simulink model "MATE_SynchronousMachine"  (R2024b)
settings: Solver=FixedStepDiscrete  StartTime=0.0  StopTime=6  FixedStep=Ts  RelTol=1e-4  EnableMultiTasking=on
PostLoadFcn:
  | Ts=25e-6;offset=4;
InitFcn:
  | Ts=25e-6;offset=4;
undefined symbols (not defined in the file): DiscIntNeverNeededParam, MATE, Phase, Rsnu, Single
libraries: fl_lib x58, nesl_utility x43, ee_lib x13, simetran x5, simetranss x3, powerlib_extras x3, simulink_extras x2, simulink x2
(part 2 of 4)

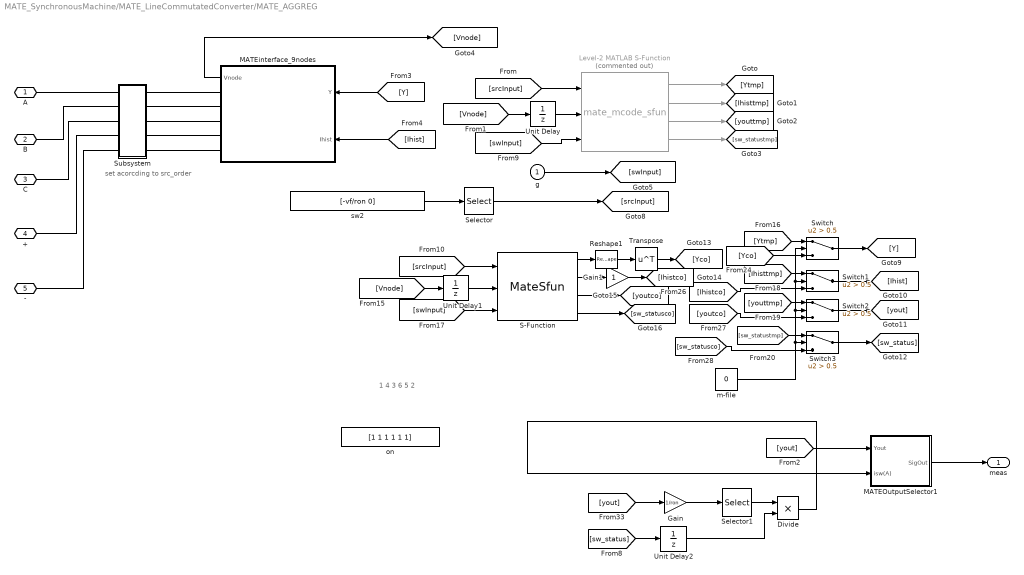
== system MATE_SynchronousMachine/MATE_LineCommutatedConverter/MATE_AGGREG ==
  note: set acorcding to src_order
  note: 1 4 3 6 5 2
  g : Inport
  Divide : Product
  Gain : Gain  Gain=1/ron
  Gain1 : Gain
  Level-2 MATLAB S-Function : M-S-Function  Commented=on  FunctionName=mate_mcode_sfun  Parameters=MATE,vf
  MATEOutputSelector1 : Subsystem
  MATEinterface_9nodes : Subsystem
  Reshape1 : Reshape  OutputDimensionality=Customize  OutputDimensions=[MATE.NumberOfNodes,MATE.NumberOfNodes]
  S-Function : S-Function  FunctionName=MateSfun  Parameters="MATERT.sizes,MATERT.As  ,MATERT.Bs,MATERT.Cs,MATERT.Ds,MATERT.Rsw,MATERT.SwType,MATERT.DISC,MATERT.h,MATERT.U0,MATERT.X0,vf"  SFunctionDeploymentMode=off  EnableBusSupport=off
  Selector : Selector  InputPortWidth=2  IndexOptions=Index vector (dialog)  Indices="[1 1 1 1 1 1  2 2 2 2 2]"  OutputSizes=1
  Selector1 : Selector  InputPortWidth=11  IndexOptions=Index vector (dialog)  Indices=[1 2 3 4 5 6]  OutputSizes=1
  Subsystem : Subsystem
  Switch{,1..3} (4 alike) : Switch  Criteria=u2 > Threshold  Threshold=0.5  SaturateOnIntegerOverflow=off  InputSameDT=off
  Transpose : Math  Operator=transpose
  Unit Delay : UnitDelay  SampleTime=Ts  HasFrameUpgradeWarning=on
  Unit Delay1 : UnitDelay  SampleTime=Ts  HasFrameUpgradeWarning=on
  Unit Delay2 : UnitDelay  SampleTime=Ts  HasFrameUpgradeWarning=on
  m-file : Constant  Value=0
  on : Constant  Value=[1 1 1 1 1 1]
  sw2 : Constant  Value=[-vf/ron 0]
  A : PMIOPort  Side=Left
  B : PMIOPort  Port=2  Side=Left
  C : PMIOPort  Port=3  Side=Left
  + : PMIOPort  Port=4  Side=Right
  - : PMIOPort  Port=5  Side=Right
  meas : Outport
  wires:
  m-file/1 -> Switch3/2, Switch/2, Switch1/2, Switch2/2
  Level-2 MATLAB S-Function/1 -> [Ytmp]
  Unit Delay/1 -> Level-2 MATLAB S-Function/2
  [swInput] -> S-Function/3
  S-Function/3 -> [youtco]
  Level-2 MATLAB S-Function/2 -> [Ihisttmp]
  Level-2 MATLAB S-Function/3 -> [youttmp]
  [youtco] -> Switch2/3
  [sw_statustmp] -> Switch3/1
  [Vnode] -> Unit Delay1/1
  [youttmp] -> Switch2/1
  [srcInput] -> Level-2 MATLAB S-Function/1
  Gain1/1 -> [Ihistco]
  [Ihistco] -> Switch1/3
  [Ytmp] -> Switch/1
  [Ihist] -> MATEinterface_9nodes/2(Ihist)
  [Vnode] -> Unit Delay/1
  [srcInput] -> S-Function/1
  Unit Delay1/1 -> S-Function/2
  S-Function/1 -> Reshape1/1
  S-Function/2 -> Gain1/1
  Switch2/1 -> [yout]
  Transpose/1 -> [Yco]
  Reshape1/1 -> Transpose/1
  S-Function/4 -> [sw_statusco]
  Switch/1 -> [Y]
  [Ihisttmp] -> Switch1/1
  [sw_statusco] -> Switch3/3
  MATEinterface_9nodes/1(Vnode) -> [Vnode]
  [swInput] -> Level-2 MATLAB S-Function/3
  [Yco] -> Switch/3
  Switch1/1 -> [Ihist]
  [Y] -> MATEinterface_9nodes/1(Y)
  Switch3/1 -> [sw_status]
  Level-2 MATLAB S-Function/4 -> [sw_statustmp]
  sw2/1 -> Selector/1
  Selector/1 -> [srcInput]
  Divide/1 -> MATEOutputSelector1/2(isw(A))
  Selector1/1 -> Divide/1
  [sw_status] -> Unit Delay2/1
  [yout] -> MATEOutputSelector1/1(Yout)
  Gain/1 -> Selector1/1
  Unit Delay2/1 -> Divide/2
  [yout] -> Gain/1
  MATEOutputSelector1/1(SigOut) -> meas/1
  g/1 -> [swInput]
  connections:
  Subsystem/RConn1 -- MATEinterface_9nodes/RConn1
  B/RConn1 -- Subsystem/LConn2
  A/RConn1 -- Subsystem/LConn1
  C/RConn1 -- Subsystem/LConn3
  +/RConn1 -- Subsystem/LConn4
  -/RConn1 -- Subsystem/LConn5
  Subsystem/RConn2 -- MATEinterface_9nodes/RConn2
  Subsystem/RConn3 -- MATEinterface_9nodes/RConn3
  Subsystem/RConn4 -- MATEinterface_9nodes/RConn4
  Subsystem/RConn5 -- MATEinterface_9nodes/RConn5

== system MATE_SynchronousMachine/Mesure et visualisation/Discrete Mean value ==
  In : Inport
  Constant : Constant  Value=Vinit  SampleTime=Ts
  Discrete Variable Transport Delay : powerlib_extras/Discrete  Control Blocks/Discrete Variable Transport Delay  MaxDelay=Delay+Ts  InitialValue=0  Ts=Ts
  Gain : Gain  Gain=K1  SaturateOnIntegerOverflow=on  OutDataTypeStr=Inherit: Same as input  ParamDataTypeStr=Inherit: Same as input
  Gain1 : Gain  Gain=K2  SaturateOnIntegerOverflow=on  OutDataTypeStr=Inherit: Same as input  ParamDataTypeStr=Inherit: Same as input
  Integ4 : DiscreteIntegrator  IntegratorMethod=Integration: Trapezoidal  SampleTime=Ts  ICPrevOutput=DiscIntNeverNeededParam  ICPrevScaledInput=DiscIntNeverNeededParam
  K1 : Constant  Value=Delay  SampleTime=Ts
  K2 : Constant  Value=Freq  SampleTime=Ts
  Product : Product  InputSameDT=on  SaturateOnIntegerOverflow=on  OutDataTypeStr=Inherit: Same as first input
  Step : Step  Time=1/Freq  SampleTime=Ts
  Sum1 : Sum  Inputs=+-  InputSameDT=on  SaturateOnIntegerOverflow=on  OutDataTypeStr=Inherit: Same as first input
  Sum5 : Sum  InputSameDT=on  SaturateOnIntegerOverflow=on  OutDataTypeStr=Inherit: Same as first input
  Sum7 : Sum  Inputs=-+  InputSameDT=on  SaturateOnIntegerOverflow=on  OutDataTypeStr=Inherit: Same as first input
  Switch : Switch  Threshold=0.5  SaturateOnIntegerOverflow=off
  Unit Delay : UnitDelay  SampleTime=Ts  HasFrameUpgradeWarning=on
  Mean : Outport  VectorParamsAs1DForOutWhenUnconnected=off
  wires:
  Product/1 -> Sum5/1  "Mean value"
  Sum7/1 -> Product/1
  Integ4/1 -> Discrete Variable Transport Delay/1, Sum7/2
  K2/1 -> Product/2
  In/1 -> Integ4/1, Gain1/1, Unit Delay/1  "In"
  Sum5/1 -> Switch/1
  Step/1 -> Switch/2
  Constant/1 -> Switch/3
  Switch/1 -> Mean/1
  Discrete Variable Transport Delay/1 -> Sum7/1
  K1/1 -> Discrete Variable Transport Delay/2
  Gain1/1 -> Sum1/1
  Unit Delay/1 -> Gain/1
  Gain/1 -> Sum1/2
  Sum1/1 -> Sum5/2  "Correction"

== system MATE_SynchronousMachine/turbine1/Hydraulic Turbine and Governor ==
  wref : Inport
  Pref : Inport  Port=2
  we : Inport  Port=3
  Pe0 : Inport  Port=4
  dw : Inport  Port=5
  Model : Subsystem  mask(Discrete Hydraulic Turbine and Governor){sm=sm, gate=gate, reg=reg, hyd=hyd, dref=dref, po=po, Ts=Ts}
      mask prompts: sm "Servo-motor [ Ka()  Ta(sec) ]:"; gate "Gate opening limits [ gmin,gmax(pu)    vgmin,vgmax(pu/s) ]:"; reg "Permanent droop and regulator  [ Rp() Kp() Ki() Kd() Td(s) ]:"; hyd "Hydraulic turbine [ beta()  Tw(sec) ]:"; dref "Droop reference (0=power error, 1=gate opening):"; po "Initial mechanical power (pu):"; Ts "Sample time:"
      mask help:
      | Implements a discrete hydraulic turbine combined to a discrete PID governor system.
      |
      | 1st input: desired speed (p.u.);
      | 2nd input: desired electrical power (p.u.);
      | 3rd input: synchronous machine's actual speed (p.u., measurement output 13 of SM block);
      | 4th input: synchronous machine's actual electrical power (p.u., measurement output 14 of SM block);
      | 5th input: synchronous machine's actual speed deviation with respect to nominal (%, measurement output 15 of SM block);
      |
      | 1st output: mechanical power to be applied to the Synchronous Machine block's 1st input (p.u.);
      | 2nd output: gate opening (p.u.).
      mask init:
      | ka=sm(1);ta=sm(2);gmin=gate(1);gmax=gate(2);vgmin=gate(3);vgmax=gate(4);Rp=reg(1);kp=reg(2);ki=reg(3);kd=reg(4);td=reg(5);beta=hyd(1);tw=hyd(2);go=po*(gmax-gmin);
      mask Help: helpview(psbhelp);
  Pm : Outport  InitialOutput=0  VectorParamsAs1DForOutWhenUnconnected=off
  gate : Outport  Port=2  InitialOutput=0  VectorParamsAs1DForOutWhenUnconnected=off
  wires:
  wref/1 -> Model/1(wref)
  Pref/1 -> Model/2(Pref)
  we/1 -> Model/3(we)
  Pe0/1 -> Model/4(Pe)
  dw/1 -> Model/5(dw)
  Model/2(gate) -> gate/1
  Model/1(Pm) -> Pm/1

== system MATE_SynchronousMachine/turbine1/Mechanical model ==
  Te : Inport  PortDimensions=1
  Pin : Inport  Port=2
  1 ----- J : Gain  Gain=1/J  SaturateOnIntegerOverflow=on  OutDataTypeStr=Inherit: Same as input  ParamDataTypeStr=Inherit: Same as input
  Delay Prediction : Subsystem
  Divide : Product  Inputs=/*
  F : Gain  Gain=F  SaturateOnIntegerOverflow=on  OutDataTypeStr=Inherit: Same as input  ParamDataTypeStr=Inherit: Same as input
  Rotor speed deviation (dw) : DiscreteIntegrator  InitialCondition=fo*2*pi  SampleTime=Ts  ICPrevOutput=DiscIntNeverNeededParam  ICPrevScaledInput=DiscIntNeverNeededParam
  Sum2 : Sum  Inputs=+--  InputSameDT=on  SaturateOnIntegerOverflow=on  OutDataTypeStr=Inherit: Same as first input
  wmec : Outport  InitialOutput=0
  delta_wm : Outport  Port=2  InitialOutput=0
  wires:
  Rotor speed deviation (dw)/1 -> delta_wm/1, F/1, Divide/1, wmec/1, Delay Prediction/1(in)  "dw"
  1 ----- J/1 -> Rotor speed deviation (dw)/1
  Divide/1 -> Sum2/1
  Te/1 -> Sum2/2  "Te"
  F/1 -> Sum2/3
  Sum2/1 -> 1 ----- J/1
  Pin/1 -> Divide/2  "Pm"

== system MATE_SynchronousMachine/Command/Regulateur de courant/Discrete 1st-Order Filter ==
  In : Inport
  Discrete State-Space : DiscreteStateSpace  A=Ad  B=Bd  C=Cd  D=Dd  InitialCondition=x0d  SampleTime=Ts
  Out : Outport  InitialOutput=0  VectorParamsAs1DForOutWhenUnconnected=off
  wires:
  In/1 -> Discrete State-Space/1
  Discrete State-Space/1 -> Out/1

== system MATE_SynchronousMachine/Command/Regulateur de courant/Discrete PI Controller1 ==
  Error : Inport  SampleTime=Ts
  Discrete-Time Integrator : DiscreteIntegrator  InitialCondition=Init  SampleTime=Ts  LimitOutput=on  UpperSaturationLimit=UpperLimit  LowerSaturationLimit=LowerLimit  ICPrevOutput=DiscIntNeverNeededParam  ICPrevScaledInput=DiscIntNeverNeededParam
  Kp4 : Gain  Gain=Kp  SaturateOnIntegerOverflow=on  SampleTime=Ts  OutDataTypeStr=Inherit: Same as input  ParamDataTypeStr=Inherit: Same as input
  Kp5 : Gain  Gain=Ki  SaturateOnIntegerOverflow=on  SampleTime=Ts  OutDataTypeStr=Inherit: Same as input  ParamDataTypeStr=Inherit: Same as input
  Saturation2 : Saturate  UpperLimit=UpperLimit  LowerLimit=LowerLimit  SampleTime=Ts
  Sum6 : Sum  InputSameDT=on  SaturateOnIntegerOverflow=on  SampleTime=Ts  OutDataTypeStr=Inherit: Same as first input
  Zero-Order Hold : ZeroOrderHold  SampleTime=Ts
  Out : Outport  SampleTime=Ts  InitialOutput=0  VectorParamsAs1DForOutWhenUnconnected=off
  wires:
  Zero-Order Hold/1 -> Sum6/1
  Saturation2/1 -> Out/1
  Discrete-Time Integrator/1 -> Sum6/2
  Kp4/1 -> Zero-Order Hold/1
  Kp5/1 -> Discrete-Time Integrator/1
  Sum6/1 -> Saturation2/1
  Error/1 -> Kp5/1, Kp4/1

== system MATE_SynchronousMachine/Command/Regulateur de tension (Mode automatique)/Discrete PI Controller1 ==
  Error : Inport  SampleTime=Ts
  Discrete-Time Integrator : DiscreteIntegrator  InitialCondition=Init  SampleTime=Ts  LimitOutput=on  UpperSaturationLimit=UpperLimit  LowerSaturationLimit=LowerLimit  ICPrevOutput=DiscIntNeverNeededParam  ICPrevScaledInput=DiscIntNeverNeededParam
  Kp4 : Gain  Gain=Kp  SaturateOnIntegerOverflow=on  SampleTime=Ts  OutDataTypeStr=Inherit: Same as input  ParamDataTypeStr=Inherit: Same as input
  Kp5 : Gain  Gain=Ki  SaturateOnIntegerOverflow=on  SampleTime=Ts  OutDataTypeStr=Inherit: Same as input  ParamDataTypeStr=Inherit: Same as input
  Saturation2 : Saturate  UpperLimit=UpperLimit  LowerLimit=LowerLimit  SampleTime=Ts
  Sum6 : Sum  InputSameDT=on  SaturateOnIntegerOverflow=on  SampleTime=Ts  OutDataTypeStr=Inherit: Same as first input
  Zero-Order Hold : ZeroOrderHold  SampleTime=Ts
  Out : Outport  SampleTime=Ts  InitialOutput=0  VectorParamsAs1DForOutWhenUnconnected=off
  wires:
  Zero-Order Hold/1 -> Sum6/1
  Saturation2/1 -> Out/1
  Discrete-Time Integrator/1 -> Sum6/2
  Kp4/1 -> Zero-Order Hold/1
  Kp5/1 -> Discrete-Time Integrator/1
  Sum6/1 -> Saturation2/1
  Error/1 -> Kp5/1, Kp4/1

== system MATE_SynchronousMachine/Command/Regulateur de tension (Mode automatique)/Discrete 3-phase Positive-Sequence Fundamental Value ==
  note: Discrete Measurement - Positive-sequence Fundamental Value
  abc : Inport  PortDimensions=3
  Cartesian to Polar : simulink_extras/Transformations/Cartesian to Polar
  Demux : Demux  Outputs=3
      settings: DisplayOption=none
  Discrete Mean value1 : Subsystem  mask(Discrete Mean value){Freq=Freq, Vinit=Real_Init, Ts=Ts}
      mask prompts: Freq "Fundamental frequency (Hz):"; Vinit "Initial input (DC component):"; Ts "Sample time:"
      mask help: Compute the mean value of the input signal over a running window of one cycle of the specified fundamental frequency.
      mask init: same as MATE_SynchronousMachine/Mesure et visualisation/Discrete Mean value
      mask Display: disp('Mean\n(discrete)')
  Discrete Mean value3 : Subsystem  mask(Discrete Mean value){Freq=Freq, Vinit=Imag_Init, Ts=Ts}
      mask prompts: Freq "Fundamental frequency (Hz):"; Vinit "Initial input (DC component):"; Ts "Sample time:"
      mask help: Compute the mean value of the input signal over a running window of one cycle of the specified fundamental frequency.
      mask init: same as MATE_SynchronousMachine/Mesure et visualisation/Discrete Mean value
      mask Display: disp('Mean\n(discrete)')
  Gain : Gain  Gain=2*pi*Freq  SaturateOnIntegerOverflow=on  OutDataTypeStr=Inherit: Same as input  ParamDataTypeStr=Inherit: Same as input
  Mux : Mux  Inputs=2
  Rad->Deg. : Gain  Gain=180/pi  SaturateOnIntegerOverflow=on  OutDataTypeStr=Inherit: Same as input  ParamDataTypeStr=Inherit: Same as input
  Terminator : Terminator
  Trigonometric Function : Trigonometry
  Trigonometric Function1 : Trigonometry  Operator=cos
  abc_to_dq0 Transformation : Subsystem  mask(abc to dq0 Transformation){}
      mask help: Perform a Park transformation from the three-phase (abc) reference frame to the dq0 reference frame.
      mask init:
      | power_initmask();
      mask Help: helpview(psbhelp);
      mask Display: disp('')
  t : DigitalClock  SampleTime=Ts
  Mag : Outport  VectorParamsAs1DForOutWhenUnconnected=off
  Phase : Outport  Port=2  VectorParamsAs1DForOutWhenUnconnected=off
  wires:
  Cartesian to Polar/2 -> Rad->Deg./1
  Cartesian to Polar/1 -> Mag/1
  Gain/1 -> Trigonometric Function1/1, Trigonometric Function/1
  t/1 -> Gain/1
  abc/1 -> abc_to_dq0 Transformation/1(abc)
  Mux/1 -> abc_to_dq0 Transformation/2(sin_cos)
  Discrete Mean value1/1(Mean) -> Cartesian to Polar/1  "Real"
  Rad->Deg./1 -> Phase/1
  Discrete Mean value3/1(Mean) -> Cartesian to Polar/2  "Real"
  abc_to_dq0 Transformation/1(dq0) -> Demux/1
  Demux/3 -> Terminator/1
  Demux/2 -> Discrete Mean value3/1(In)
  Demux/1 -> Discrete Mean value1/1(In)
  Trigonometric Function/1 -> Mux/1
  Trigonometric Function1/1 -> Mux/2

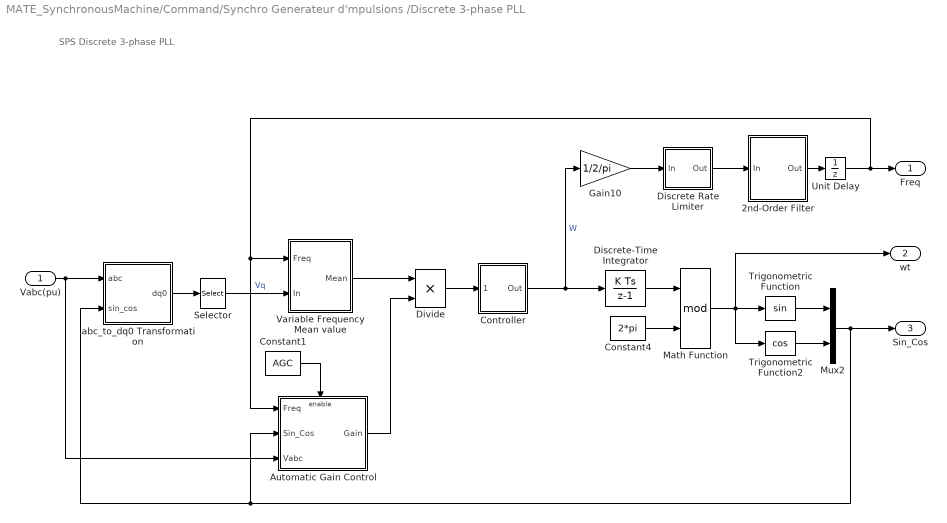
== system MATE_SynchronousMachine/Command/Synchro Generateur d'mpulsions /Discrete 3-phase PLL ==
  note: SPS Discrete 3-phase PLL
  Vabc(pu) : Inport  PortDimensions=3
  2nd-Order Filter : Subsystem  mask(Discrete 2nd-Order Filter){FilterType=Lowpass, Fo=25, Zeta=0.707, Ts=Ts, Initialize=on, Vac_Init=[0 0 Finit], Vdc_Init=Finit, PlotResponse=off, param1=[1 500 0.1]}
      mask prompts: FilterType "Filter Type:"; Fo "Cut-off frequency (Hz):"; Zeta "Damping factor Zeta ( Q = 1 / (2*Zeta) ):"; Ts "Sample time:"; Initialize "Initialize filter states"; Vac_Init "AC initial input: [ Mag  Phase(degrees)  Freq(Hz) ]"; Vdc_Init "DC Initial input:"; PlotResponse "Plot filter response"; param1 "Frequency range(Hz) : [Start  End  Inc.]"
      mask init:
      | str=sprintf(' Fo=%iHz\n\n',Fo);
      | Wo=2*pi*Fo;
      | switch FilterType
      | case 1, % Lowpass
      |        X=[0 1 2 3 4];
      |        Y=[-2 -2 -3 -4 -4];
      |        n2=0;n1=0;n0=Wo*Wo;
      |        d2=1;d1=2*Zeta*Wo;d0=Wo*Wo;
      | 	   Ystep=1;
      |  case 2,   % Highpass
      |        X=[0 1 2 3 4];
      |        Y=[-4 -4 -3 -2 -2];
      |        n2=1;n1=0;n0=0;
      |        d2=1;d1=2*Zeta*Wo;d0=Wo*Wo;
      | 	   Ystep=2;
      |     case 3,   % Bandpass
      |        X=[0 1 2 3 4 5 ];
      |        Y=[-3 -3 -2 -2 -3 -3];
      |        n2=0;n1=2*Zeta*Wo;n0=0;
      |        d2=1;d1=2*Zeta*Wo;d0=Wo*Wo;
      | 	   Ystep=3;
      |     case 4,  %Bandstop (Notch)
      |        X=[0 1 2 3 4 5 ];
      |        Y=[-2 -2 -3 -3 -2 -2];
      |        n2=1;n1=0;n0=Wo*Wo;
      |        d2=1;d1=2*Zeta*Wo;d0=Wo*Wo;
      | 	   Ystep=4;
      |     end
      | %
      | numc=[n2 n1 n0];
      | denc=[d2 d1 d0];
      | [Ac,Bc,Cc,Dc]=tf2ss(numc,denc);
      | %
      | %  Conversion to discrete transfer function
      | nstates = size(Ac,1);
      | invexp = inv(eye(nstates) - (Ts/2)*Ac);
      | Ad = invexp*(eye(nstates) + (Ts/2)*Ac);
      | Bd = invexp*Bc;
      | Cd = Cc*invexp*Ts;
      | Dd = Cc*invexp*Bc*(Ts/2) + Dc;
      | %
      | if Initialize==1  % Compute initial conditions on states
      | u1=Vac_Init(1)*exp(j*Vac_Init(2)*pi/180);
      | u2=Vdc_Init*exp(j*90*pi/180);
      | u=u1+u2;
      | u0=imag(u); % input at  t=0;
      | I=eye(size(Ac));
      | sI1=I*j*(2*pi*Vac_Init(3));
      | sI2=I*j*0;
      | x=inv(sI1-Ac)*Bc*u1 + inv(sI2-Ac)*Bc*u2;
      | x0c=imag(x);
      | x0d=(I-Ac*Ts/2)*x0c/Ts - Bc/2*u0;
      | else
      | x0d=0;
      | end
      | %
      | if PlotResponse==1 % Plot frequency and step response
      | if Zeta==1
      | 	z=1+1e-12;
      | else
      | 	z=Zeta;
      | end
      | wn=Wo;
      | t=[0:1/(z*wn)/1000:7/(z*wn)];
      | f=param1(1):param1(3):param1(2);
      | w=2*pi*f;
      | switch FilterType
      | 	case 1, % Lowpass
      | 		Ystep=wn^2*(1/wn^2+1/(4*z^2*wn^2-4*wn^2)^(1/2)*(1/(-z*wn+1/2*(4*z^2*wn^2-4*wn^2)^(1/2))*exp((-z*wn+1/2*(4*z^2*wn^2-4*wn^2)^(1/2))*t)-1/(-z*wn-1/2*(4*z^2*wn^2-4*wn^2)^(1/2))*exp((-z*wn-1/2*(4*z^2*wn^2-4*wn^2)^(1/2))*t)));
      | 		numFreq=wn^2;
      | 	case 2,   % Highpass
      | 		Ystep=-exp(-z*wn*t)/(z-1)/(z+1).*cos((-wn^2*(z-1)*(z+1))^(1/2)*t)+exp(-z*wn*t)/(z-1)/(z+1)*z^2.*cos((-wn^2*(z-1)*(z+1))^(1/2)*t)+z/wn*exp(-z*wn*t)/(z-1)/(z+1)*(wn^2-z^2*wn^2)^(1/2).*sin((-wn^2*(z-1)*(z+1))^(1/2)*t);
      | 		numFreq=-w.^2;
      | 	case 3,   % Bandpass
      | 		Ystep=2*z*wn/(4*z^2*wn^2-4*wn^2)^(1/2)*(exp((-z*wn+1/2*(4*z^2*wn^2-4*wn^2)^(1/2))*t)-exp((-z*wn-1/2*(4*z^2*wn^2-4*wn^2)^(1/2))*t));
      | 		numFreq=2*Zeta*wn.*w*j;
      | 	case 4,  %Bandstop (Notch)
      | 		Ystep=1+2*z/wn*exp(-z*wn*t)/(z-1)/(z+1)*(wn^2-z^2*wn^2)^(1/2).*sin((-wn^2*(z-1)*(z+1))^(1/2)*t);	
      | 		numFreq=wn^2-w.^2;
      | end
      | %
      | denFreq=(wn^2-w.^2) + 2*Zeta*wn*j.*w;
      | RepFreq=numFreq./denFreq;
      | Mag=abs(RepFreq);
      | Pha=angle(RepFreq)*180/pi;
      | %
      | figure(1)
      | subplot(2,1,1)
      | plot(f,Mag)
      | grid
      | title('Bode Diagram')
      | ylabel('Magnitude')
      | subplot(2,1,2)
      | plot(f,Pha)
      | ylabel('Phase (deg)')
      | xlabel('Frequency (Hz)')
      | grid
      | figure(2)
      | plot(t,real(Ystep))
      | grid
      | ylabel('Amplitude')
      | xlabel('Time (s)')
      | title('Step Response')
      | end
      mask Help: This block is part of a subset of blocks in the Extras library that does not have documentation associated with it, other than the block mask description.
      mask TypeOptions FilterType: Lowpass | Highpass | Bandpass | Bandstop (Notch)
      mask Callback Initialize: p5=get_param(gcb,'Initialize');if strcmp(p5,'on');visible={'on','on','on','on','on','on','on','on',get_param(gcb,'PlotResponse')};else;visible={'on','on','on','on','on','off','off','on',get_param(gcb,'PlotResponse')};end;set_param(gcb,'MaskVisibilities',visible)
      mask Callback PlotResponse: p8=get_param(gcb,'PlotResponse');if strcmp(p8,'on');visible={'on','on','on','on','on',get_param(gcb,'Initialize'),get_param(gcb,'Initialize'),'on','on'};else;visible={'on','on','on','on','on',get_param(gcb,'Initialize'),get_param(gcb,'Initialize'),'on','off'};end;set_param(gcb,'MaskVisibilities',visible)
      mask Display:
      | plot(X,Y);
      | disp(str);
  Automatic Gain Control : Subsystem  TreatAsAtomicUnit=on
  Constant1 : Constant  Value=AGC
  Constant4 : Constant  Value=2*pi
  Controller : Subsystem  mask(Discrete PID Controller){Kp=Kp, Ki=Ki, Kd=Kd, Par_Limits=[10000 0], Init=2*pi*Finit, Ts=Ts}
      mask prompts: Kp "Proportional gain (Kp):"; Ki "Integral gain (Ki):"; Kd "Derivative gain (Kd):"; Par_Limits "Output limits: [ Upper   Lower ]"; Init "Output initial value:"; Ts "Sample time:"
      mask help: This block implements a discrete PID controller.
      mask init:
      | UpperLimit=Par_Limits(1);
      | LowerLimit=Par_Limits(2);
      settings: OpenFcn=power_openblockproxy();
      mask Display: disp('PID');
  Discrete Rate Limiter : Subsystem  mask(Discrete Rate Limiter){R=12, F=-12, Vinit=Finit, Ts=Ts}
      mask prompts: R "Rising slew rate:"; F "Falling slew rate:"; Vinit "Initial input:"; Ts "Sample time:"
      mask init:
      | UpperLimit=R*Ts;
      | LowerLimit=F*Ts;
      mask Display: disp('Discrete\nRate\nLimiter')
  Discrete-Time Integrator : DiscreteIntegrator  InitialCondition=Phase_Init*pi/180  SampleTime=Ts  ICPrevOutput=DiscIntNeverNeededParam  ICPrevScaledInput=DiscIntNeverNeededParam
  Divide : Product
  Gain10 : Gain  Gain=1/2/pi  SaturateOnIntegerOverflow=on  OutDataTypeStr=Inherit: Same as input  ParamDataTypeStr=Inherit: Same as input
  Math Function : Math  Operator=mod  SignedPower=on
  Mux2 : Mux  Inputs=2
  Selector : Selector  InputPortWidth=3  IndexOptions=Index vector (dialog)  Indices=2  OutputSizes=1
  Trigonometric Function : Trigonometry
  Trigonometric Function2 : Trigonometry  Operator=cos
  Unit Delay : UnitDelay  InitialCondition=Finit  SampleTime=Ts  HasFrameUpgradeWarning=on
  Variable Frequency Mean value : Subsystem  mask(Discrete Variable-Frequency Mean Value){Finit=Finit, Fmin=Fmin, Vinit=0, Ts=Ts}
      mask prompts: Finit "Initial frequency (Hz):"; Fmin "Minimum frequency (Hz):"; Vinit "Initial input (DC component):"; Ts "Sample time:"
      mask help: Compute the mean value of input 2 over a running window of one cycle of frequency given by input 1.
      mask init:
      | MaxDelay=1/Fmin+Ts;
      mask Display: disp('')
  abc_to_dq0 Transformation : Subsystem  mask(abc to dq0 Transformation){}
      mask help: Perform a Park transformation from the three-phase (abc) reference frame to the dq0 reference frame.
      mask Display: disp('')
  Freq : Outport  VectorParamsAs1DForOutWhenUnconnected=off
  wt : Outport  Port=2  VectorParamsAs1DForOutWhenUnconnected=off
  Sin_Cos : Outport  Port=3  VectorParamsAs1DForOutWhenUnconnected=off
  wires:
  Selector/1 -> Variable Frequency Mean value/2(In)  "Vq"
  2nd-Order Filter/1(Out) -> Unit Delay/1
  Unit Delay/1 -> Freq/1, Variable Frequency Mean value/1(Freq), Automatic Gain Control/1(Freq)
  Discrete Rate Limiter/1(Out) -> 2nd-Order Filter/1(In)
  Gain10/1 -> Discrete Rate Limiter/1(In)
  Mux2/1 -> Sin_Cos/1, abc_to_dq0 Transformation/2(sin_cos), Automatic Gain Control/2(Sin_Cos)
  Trigonometric Function2/1 -> Mux2/2
  Trigonometric Function/1 -> Mux2/1
  Math Function/1 -> wt/1, Trigonometric Function2/1, Trigonometric Function/1
  Discrete-Time Integrator/1 -> Math Function/1
  Constant4/1 -> Math Function/2
  abc_to_dq0 Transformation/1(dq0) -> Selector/1
  Vabc(pu)/1 -> abc_to_dq0 Transformation/1(abc), Automatic Gain Control/3(Vabc)
  Controller/1(Out) -> Discrete-Time Integrator/1, Gain10/1  "W"
  Variable Frequency Mean value/1(Mean) -> Divide/1
  Automatic Gain Control/1(Gain) -> Divide/2
  Divide/1 -> Controller/1(Error)
  Constant1/1 -> Automatic Gain Control/Enable

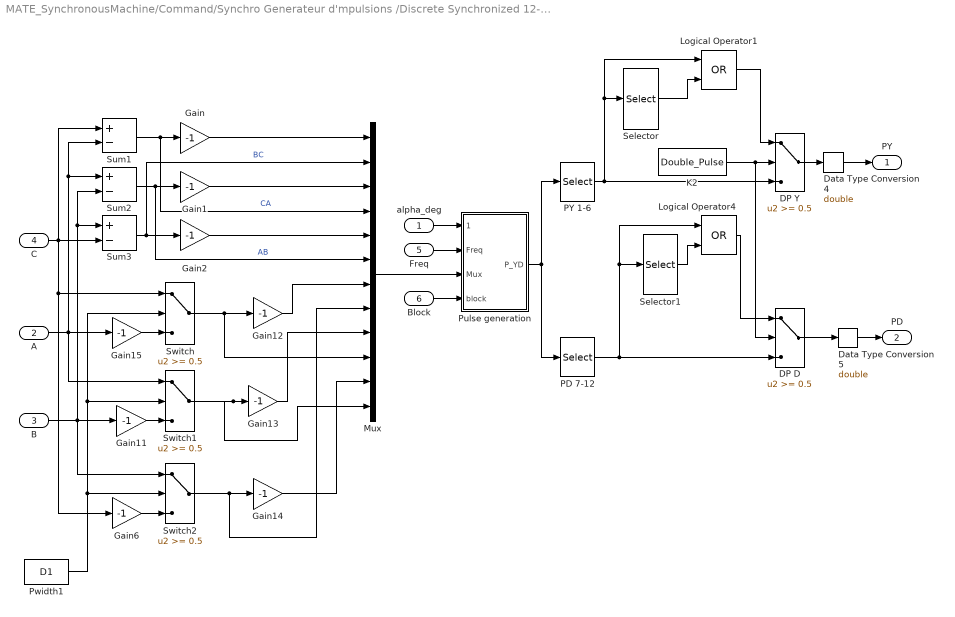
== system MATE_SynchronousMachine/Command/Synchro Generateur d'mpulsions /Discrete Synchronized 12-Pulse Generator ==
  alpha_deg : Inport
  A : Inport  Port=2
  B : Inport  Port=3
  C : Inport  Port=4
  Freq : Inport  Port=5
  Block : Inport  Port=6
  DP D : Switch  Threshold=0.5  SaturateOnIntegerOverflow=off
  DP Y : Switch  Threshold=0.5  SaturateOnIntegerOverflow=off
  Data Type Conversion4 : DataTypeConversion  OutDataTypeStr=double
  Data Type Conversion5 : DataTypeConversion  OutDataTypeStr=double
  Gain{,1..2,6,11..15} (9 alike) : Gain  Gain=-1  SaturateOnIntegerOverflow=on  OutDataTypeStr=Inherit: Same as input  ParamDataTypeStr=Inherit: Same as input
  K2 : Constant  Value=Double_Pulse
  Logical Operator1 : Logic  Operator=OR
  Logical Operator4 : Logic  Operator=OR
  Mux : Mux  Inputs=12
  PD 7-12 : Selector  InputPortWidth=12  IndexOptions=Index vector (dialog)  Indices=7:12  OutputSizes=1
  PY 1-6 : Selector  InputPortWidth=12  IndexOptions=Index vector (dialog)  Indices=1:6  OutputSizes=1
  Pulse generation : Subsystem
  Pwidth1 : Constant  Value=D1
  Selector : Selector  InputPortWidth=6  IndexOptions=Index vector (dialog)  Indices=[2 3 4 5 6 1 ]  OutputSizes=1
  Selector1 : Selector  InputPortWidth=6  IndexOptions=Index vector (dialog)  Indices=[2 3 4 5 6 1 ]  OutputSizes=1
  Sum1 : Sum  Inputs=+-  InputSameDT=on  SaturateOnIntegerOverflow=on  OutDataTypeStr=Inherit: Same as first input
  Sum2 : Sum  Inputs=+-  InputSameDT=on  SaturateOnIntegerOverflow=on  OutDataTypeStr=Inherit: Same as first input
  Sum3 : Sum  Inputs=+-  InputSameDT=on  SaturateOnIntegerOverflow=on  OutDataTypeStr=Inherit: Same as first input
  Switch : Switch  Threshold=0.5  SaturateOnIntegerOverflow=off  InputSameDT=off
  Switch1 : Switch  Threshold=0.5  SaturateOnIntegerOverflow=off  InputSameDT=off
  Switch2 : Switch  Threshold=0.5  SaturateOnIntegerOverflow=off  InputSameDT=off
  PY : Outport  InitialOutput=0  VectorParamsAs1DForOutWhenUnconnected=off
  PD : Outport  Port=2  InitialOutput=0  VectorParamsAs1DForOutWhenUnconnected=off
  wires:
  Pulse generation/1(P_YD) -> PY 1-6/1, PD 7-12/1
  Freq/1 -> Pulse generation/2(Freq)
  alpha_deg/1 -> Pulse generation/1(alpha_deg)
  Logical Operator1/1 -> DP Y/1
  Selector/1 -> Logical Operator1/2
  PY 1-6/1 -> DP Y/3, Selector/1, Logical Operator1/1
  Logical Operator4/1 -> DP D/1
  Selector1/1 -> Logical Operator4/2
  PD 7-12/1 -> Logical Operator4/1, Selector1/1, DP D/3
  K2/1 -> DP Y/2, DP D/2
  Block/1 -> Pulse generation/4(block)
  DP Y/1 -> Data Type Conversion4/1
  Data Type Conversion4/1 -> PY/1
  DP D/1 -> Data Type Conversion5/1
  Data Type Conversion5/1 -> PD/1
  Pwidth1/1 -> Switch2/2, Switch1/2, Switch/2
  Gain14/1 -> Mux/11
  Gain13/1 -> Mux/9
  Gain12/1 -> Mux/7
  Gain6/1 -> Switch2/3
  Gain11/1 -> Switch1/3
  Gain15/1 -> Switch/3
  Switch/1 -> Mux/10, Gain12/1
  Switch2/1 -> Mux/8, Gain14/1
  Switch1/1 -> Mux/12, Gain13/1
  Mux/1 -> Pulse generation/3(Mux)
  Gain2/1 -> Mux/5
  Gain1/1 -> Mux/3
  Gain/1 -> Mux/1
  Sum1/1 -> Gain/1, Mux/4  "CA"
  Sum2/1 -> Gain1/1, Mux/6  "AB"
  Sum3/1 -> Gain2/1, Mux/2  "BC"
  C/1 -> Switch/1, Gain6/1, Sum1/1, Sum3/2
  A/1 -> Switch1/1, Gain15/1, Sum2/1, Sum1/2
  B/1 -> Switch2/1, Sum2/2, Sum3/1, Gain11/1

== system MATE_SynchronousMachine/MATE_LineCommutatedConverter/MATEPREP/RCsnuber ==
  Capacitor : fl_lib/Electrical/Electrical Elements/Capacitor  c=Csnu F  r=0 Ohm  g=0 1/Ohm  i_specify=off  i_priority=None  i=0 A  i_nominal_specify=off  i_nominal_value=1  i_nominal_unit=A  v_specify=off  v_priority=None  v=0 V  v_nominal_specify=off  v_nominal_value=1  v_nominal_unit=V  vc_specify=off  vc_priority=High  vc=0 V  vc_nominal_specify=off  vc_nominal_value=1  vc_nominal_unit=V
  Resistor : fl_lib/Electrical/Electrical Elements/Resistor  R=Rsnu Ohm  i_specify=off  i_priority=None  i=0 A  i_nominal_specify=off  i_nominal_value=1  i_nominal_unit=A  v_specify=off  v_priority=None  v=0 V  v_nominal_specify=off  v_nominal_value=1  v_nominal_unit=V
  + : PMIOPort  Side=Left
  - : PMIOPort  Port=2  Side=Right
  connections:
  Resistor/LConn1 -- Capacitor/RConn1
  Capacitor/LConn1 -- +/RConn1
  Resistor/RConn1 -- -/RConn1

== system MATE_SynchronousMachine/MATE_LineCommutatedConverter/MATEPREP/RCsnuber1 ==
  Capacitor : fl_lib/Electrical/Electrical Elements/Capacitor  c=Csnu F  r=0 Ohm  g=0 1/Ohm  i_specify=off  i_priority=None  i=0 A  i_nominal_specify=off  i_nominal_value=1  i_nominal_unit=A  v_specify=off  v_priority=None  v=0 V  v_nominal_specify=off  v_nominal_value=1  v_nominal_unit=V  vc_specify=off  vc_priority=High  vc=0 V  vc_nominal_specify=off  vc_nominal_value=1  vc_nominal_unit=V
  Resistor : fl_lib/Electrical/Electrical Elements/Resistor  R=Rsnu Ohm  i_specify=off  i_priority=None  i=0 A  i_nominal_specify=off  i_nominal_value=1  i_nominal_unit=A  v_specify=off  v_priority=None  v=0 V  v_nominal_specify=off  v_nominal_value=1  v_nominal_unit=V
  + : PMIOPort  Side=Left
  - : PMIOPort  Port=2  Side=Right
  connections:
  Resistor/RConn1 -- -/RConn1
  Capacitor/LConn1 -- +/RConn1
  Resistor/LConn1 -- Capacitor/RConn1

== system MATE_SynchronousMachine/MATE_LineCommutatedConverter/MATEPREP/RCsnuber2 ==
  Capacitor : fl_lib/Electrical/Electrical Elements/Capacitor  c=Csnu F  r=0 Ohm  g=0 1/Ohm  i_specify=off  i_priority=None  i=0 A  i_nominal_specify=off  i_nominal_value=1  i_nominal_unit=A  v_specify=off  v_priority=None  v=0 V  v_nominal_specify=off  v_nominal_value=1  v_nominal_unit=V  vc_specify=off  vc_priority=High  vc=0 V  vc_nominal_specify=off  vc_nominal_value=1  vc_nominal_unit=V
  Resistor : fl_lib/Electrical/Electrical Elements/Resistor  R=Rsnu Ohm  i_specify=off  i_priority=None  i=0 A  i_nominal_specify=off  i_nominal_value=1  i_nominal_unit=A  v_specify=off  v_priority=None  v=0 V  v_nominal_specify=off  v_nominal_value=1  v_nominal_unit=V
  + : PMIOPort  Side=Left
  - : PMIOPort  Port=2  Side=Right
  connections:
  Resistor/LConn1 -- Capacitor/RConn1
  Capacitor/LConn1 -- +/RConn1
  Resistor/RConn1 -- -/RConn1

== system MATE_SynchronousMachine/MATE_LineCommutatedConverter/MATEPREP/RCsnuber3 ==
  Capacitor : fl_lib/Electrical/Electrical Elements/Capacitor  c=Csnu F  r=0 Ohm  g=0 1/Ohm  i_specify=off  i_priority=None  i=0 A  i_nominal_specify=off  i_nominal_value=1  i_nominal_unit=A  v_specify=off  v_priority=None  v=0 V  v_nominal_specify=off  v_nominal_value=1  v_nominal_unit=V  vc_specify=off  vc_priority=High  vc=0 V  vc_nominal_specify=off  vc_nominal_value=1  vc_nominal_unit=V
  Resistor : fl_lib/Electrical/Electrical Elements/Resistor  R=Rsnu Ohm  i_specify=off  i_priority=None  i=0 A  i_nominal_specify=off  i_nominal_value=1  i_nominal_unit=A  v_specify=off  v_priority=None  v=0 V  v_nominal_specify=off  v_nominal_value=1  v_nominal_unit=V
  + : PMIOPort  Side=Left
  - : PMIOPort  Port=2  Side=Right
  connections:
  Resistor/RConn1 -- -/RConn1
  Capacitor/LConn1 -- +/RConn1
  Resistor/LConn1 -- Capacitor/RConn1

== system MATE_SynchronousMachine/MATE_LineCommutatedConverter/MATEPREP/RCsnuber4 ==
  Capacitor : fl_lib/Electrical/Electrical Elements/Capacitor  c=Csnu F  r=0 Ohm  g=0 1/Ohm  i_specify=off  i_priority=None  i=0 A  i_nominal_specify=off  i_nominal_value=1  i_nominal_unit=A  v_specify=off  v_priority=None  v=0 V  v_nominal_specify=off  v_nominal_value=1  v_nominal_unit=V  vc_specify=off  vc_priority=High  vc=0 V  vc_nominal_specify=off  vc_nominal_value=1  vc_nominal_unit=V
  Resistor : fl_lib/Electrical/Electrical Elements/Resistor  R=Rsnu Ohm  i_specify=off  i_priority=None  i=0 A  i_nominal_specify=off  i_nominal_value=1  i_nominal_unit=A  v_specify=off  v_priority=None  v=0 V  v_nominal_specify=off  v_nominal_value=1  v_nominal_unit=V
  + : PMIOPort  Side=Left
  - : PMIOPort  Port=2  Side=Right
  connections:
  Resistor/RConn1 -- -/RConn1
  Capacitor/LConn1 -- +/RConn1
  Resistor/LConn1 -- Capacitor/RConn1

== system MATE_SynchronousMachine/MATE_LineCommutatedConverter/MATEPREP/RCsnuber5 ==
  Capacitor : fl_lib/Electrical/Electrical Elements/Capacitor  c=Csnu F  r=0 Ohm  g=0 1/Ohm  i_specify=off  i_priority=None  i=0 A  i_nominal_specify=off  i_nominal_value=1  i_nominal_unit=A  v_specify=off  v_priority=None  v=0 V  v_nominal_specify=off  v_nominal_value=1  v_nominal_unit=V  vc_specify=off  vc_priority=High  vc=0 V  vc_nominal_specify=off  vc_nominal_value=1  vc_nominal_unit=V
  Resistor : fl_lib/Electrical/Electrical Elements/Resistor  R=Rsnu Ohm  i_specify=off  i_priority=None  i=0 A  i_nominal_specify=off  i_nominal_value=1  i_nominal_unit=A  v_specify=off  v_priority=None  v=0 V  v_nominal_specify=off  v_nominal_value=1  v_nominal_unit=V
  + : PMIOPort  Side=Left
  - : PMIOPort  Port=2  Side=Right
  connections:
  Resistor/LConn1 -- Capacitor/RConn1
  Capacitor/LConn1 -- +/RConn1
  Resistor/RConn1 -- -/RConn1

== system MATE_SynchronousMachine/MATE_LineCommutatedConverter/MATE_AGGREG/MATEOutputSelector1 ==
  Yout : Inport
  isw(A) : Inport  Port=2
  BusCreator : BusCreator  Inputs=12
  Demux : Demux  Outputs=11
  SigOut : Outport
  wires:
  isw(A)/1 -> BusCreator/12  "Switch currents(A)"
  BusCreator/1 -> SigOut/1
  Yout/1 -> Demux/1
  Demux/1 -> BusCreator/1  "Leg A upperThy Voltage(V)"
  Demux/2 -> BusCreator/2  "Leg A lowerThy Voltage(V)"
  Demux/3 -> BusCreator/3  "Leg B upperThy Voltage(V)"
  Demux/4 -> BusCreator/4  "Leg B lowerThy Voltage(V)"
  Demux/5 -> BusCreator/5  "Leg C upperThy Voltage(V)"
  Demux/6 -> BusCreator/6  "Leg C lowerThy Voltage(V)"
  Demux/7 -> BusCreator/7  "+ terminal voltage (V)"
  Demux/8 -> BusCreator/8  "- terminal voltage (V)"
  Demux/9 -> BusCreator/9  "A terminal voltage (V)"
  Demux/10 -> BusCreator/10  "B terminal voltage (V)"
  Demux/11 -> BusCreator/11  "C terminal voltage (V)"

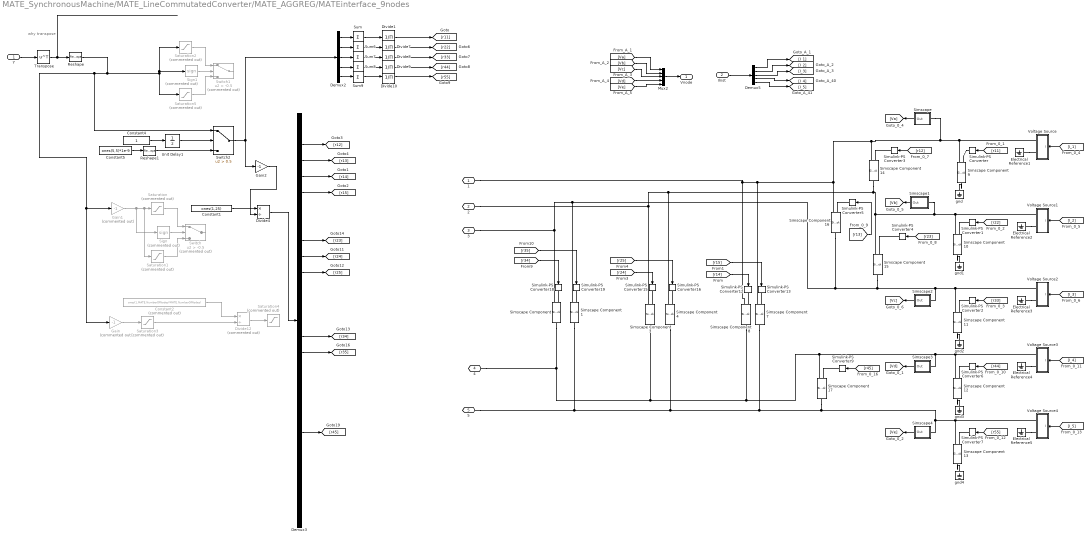
== system MATE_SynchronousMachine/MATE_LineCommutatedConverter/MATE_AGGREG/MATEinterface_9nodes ==
  note: why transpose
  Y : Inport
  Ihist : Inport  Port=2
  Constant1 : Constant  Value=ones(1,25)
  Constant2 : Constant  Commented=on  Value=ones(1,MATE.NumberOfNodes*MATE.NumberOfNodes)
  Constant4 : Constant
  Constant5 : Constant  Value=ones(5,5)*1e-9
  Demux2 : Demux  Outputs=[5 5 5 5 5]
      settings: DisplayOption=none
  Demux3 : Demux  Outputs=25
      settings: DisplayOption=none
  Demux5 : Demux  Outputs=[1 1 1 1 1]
      settings: DisplayOption=none
  Divide{1,7..10} (5 alike) : Product  Inputs=/
  Divide12 : Product  Commented=on  Inputs=*/  CollapseMode=Specified dimension
  Divide4 : Product  Inputs=*/  CollapseMode=Specified dimension
  Electrical Reference{1..5} (5 alike) : fl_lib/Electrical/Electrical Elements/Electrical Reference
  Gain : Gain  Commented=on  Gain=-1
  Gain1 : Gain  Commented=on  Gain=-1
  Gain2 : Gain  Gain=-1
  Mux2 : Mux  Inputs=[1 1 1 1 1]
  Reshape : Reshape
  Reshape1 : Reshape
  Saturation : Saturate  Commented=on  UpperLimit=1e12  LowerLimit=1e-12
  Saturation1 : Saturate  Commented=on  UpperLimit=-1e-12  LowerLimit=-1e12
  Saturation2 : Saturate  Commented=on  UpperLimit=1e12  LowerLimit=1e-12
  Saturation3 : Saturate  Commented=on  UpperLimit=1e15  LowerLimit=-1e15
  Saturation4 : Saturate  Commented=on  UpperLimit=1e15  LowerLimit=-1e15
  Saturation5 : Saturate  Commented=on  UpperLimit=-1e-12  LowerLimit=-1e12
  Sign : Signum  Commented=on
  Sign1 : Signum  Commented=on
  Simscape : Subsystem
      mask Display: disp('V')
  Simscape Component{,1,3..4,7..17} (15 alike) : SimscapeComponentBlock  SourceFile=variable_resistor_unlimited  ComponentPath=variable_resistor_unlimited  ComponentVariants="[\"variable_resistor_unlimited\"]"  ComponentVariantNames="[\"variable_resistor_unlimited\"]"  ClassName=variable_resistor_unlimited  SchemaVersion=1  R0=0 Ohm  Rmaxp=1e9 Ohm  Rmaxn=-1e9 Ohm  Rminp=1e-9 Ohm  Rminn=-1e-9 Ohm  i_specify=off  i_priority=None  i=0 A  i_nominal_specify=off  i_nominal_value=1  i_nominal_unit=A  v_specify=off  v_priority=None  v=0 V  v_nominal_specify=off  v_nominal_value=1  v_nominal_unit=V
      settings: CopyFcn=simscape.engine.sli.internal.componentblockcallback(gcbh,'COPY')  PreCopyFcn=simscape.engine.sli.internal.componentblockcallback(gcbh,'PRECOPY')  PreDeleteFcn=simscape.engine.sli.internal.componentblockcallback(gcbh,'PREDELETE')  InternalSimscapePortConfiguration="{\"Bottom\":[],\"Left\":[{\"id\":\"R\",\"label\":\"R\",\"type\":\"input\"},{\"id\":\"p\",\"label\":\"+\",\"type\":\"foundation.electrical.electrical\"}],\"Right\":[{\"id\":\"n\",\"label\":\"-\",\"type\":\"foundation.electrical.electrical\"}],\"Top\":[]}"
      mask Type: Variable Resistor
  Simscape1 : Subsystem
      mask Display: disp('V')
  Simscape2 : Subsystem
      mask Display: disp('V')
  Simscape3 : Subsystem
      mask Display: disp('V')
  Simscape4 : Subsystem
      mask Display: disp('V')
  Simulink-PS Converter{,1..7,9,12..13,15..16,18..19} (15 alike) : nesl_utility/Simulink-PS Converter  PhysicalDomain=network_engine_domain  SubClassName=ps_input  LeftPortType=input  RightPortType=output  PseudoPeriodic=off  Frequencies=[]  NoiseDistribution=none  NoiseParameters=[]  Unit=1  AffineConversion=off  FilteringAndDerivatives=provide  SimscapeFilterOrder=1  InputFilterTimeConstant=0.001  UdotUserProvided=0
  Sum{,6..9} (5 alike) : Sum  Inputs=+
  Switch : Switch  Commented=on  Criteria=u2 > Threshold  Threshold=-0.5  SaturateOnIntegerOverflow=off  InputSameDT=off
  Switch1 : Switch  Commented=on  Criteria=u2 > Threshold  Threshold=-0.5  SaturateOnIntegerOverflow=off  InputSameDT=off
  Switch2 : Switch  Criteria=u2 > Threshold  Threshold=0.5  SaturateOnIntegerOverflow=off  InputSameDT=off
  Transpose : Math  Operator=transpose
  Unit Delay1 : UnitDelay  SampleTime=Ts  HasFrameUpgradeWarning=on
  Voltage Source : Subsystem
  Voltage Source1 : Subsystem
  Voltage Source2 : Subsystem
  Voltage Source3 : Subsystem
  Voltage Source4 : Subsystem
  gnd{,1..4} (5 alike) : fl_lib/Electrical/Electrical Elements/Electrical Reference
  1 : PMIOPort  Side=Right
  2 : PMIOPort  Port=2  Side=Right
  3 : PMIOPort  Port=3  Side=Right
  4 : PMIOPort  Port=4  Side=Right
  5 : PMIOPort  Port=5  Side=Right
  Vnode : Outport  VectorParamsAs1DForOutWhenUnconnected=off
  wires:
  [I_2] -> Voltage Source1/1(I)
  Simscape2/1(Out) -> [Vc]
  [I_3] -> Voltage Source2/1(I)
  Simscape/1(Out) -> [Va]
  Simscape1/1(Out) -> [Vb]
  [I_1] -> Voltage Source/1(I)
  Y/1 -> Transpose/1
  Transpose/1 -> Reshape/1
  [r11] -> Simulink-PS Converter/1
  Sum/1 -> Divide1/1
  Divide1/1 -> [r11]
  [r22] -> Simulink-PS Converter1/1
  [r33] -> Simulink-PS Converter2/1
  [r12] -> Simulink-PS Converter3/1
  [r23] -> Simulink-PS Converter4/1
  [r13] -> Simulink-PS Converter5/1
  Demux2/1 -> Sum/1
  Divide7/1 -> [r22]
  Sum6/1 -> Divide7/1
  Demux2/2 -> Sum6/1
  Sum7/1 -> Divide8/1
  Divide8/1 -> [r33]
  Demux2/3 -> Sum7/1
  Demux2/4 -> Sum8/1
  Divide9/1 -> [r44]
  Sum8/1 -> Divide9/1
  Sum9/1 -> Divide10/1
  Divide10/1 -> [r55]
  Demux2/5 -> Sum9/1
  [r44] -> Simulink-PS Converter6/1
  [I_4] -> Voltage Source3/1(I)
  Simscape3/1(Out) -> [Vd]
  Simscape4/1(Out) -> [Ve]
  [I_5] -> Voltage Source4/1(I)
  [r55] -> Simulink-PS Converter7/1
  [r45] -> Simulink-PS Converter9/1
  [r14] -> Simulink-PS Converter12/1
  [r15] -> Simulink-PS Converter13/1
  [r25] -> Simulink-PS Converter16/1
  [r24] -> Simulink-PS Converter15/1
  Mux2/1 -> Vnode/1
  Ihist/1 -> Demux5/1
  Demux3/2 -> [r12]
  Demux3/3 -> [r13]
  Demux3/4 -> [r14]
  Demux3/5 -> [r15]
  Gain1/1 -> Sign/1, Saturation1/1, Saturation/1
  Constant1/1 -> Divide4/1
  [r35] -> Simulink-PS Converter19/1
  [r34] -> Simulink-PS Converter18/1
  Sign/1 -> Switch/2
  Saturation/1 -> Switch/1
  Saturation1/1 -> Switch/3
  Divide12/1 -> Saturation4/1
  Saturation3/1 -> Divide12/2
  Constant2/1 -> Divide12/1
  Gain/1 -> Saturation3/1
  Saturation5/1 -> Switch1/3
  Saturation2/1 -> Switch1/1
  Sign1/1 -> Switch1/2
  Reshape/1 -> Gain1/1, Gain/1, Switch2/1, Saturation2/1, Sign1/1, Saturation5/1
  Unit Delay1/1 -> Switch2/2
  Constant4/1 -> Unit Delay1/1
  Reshape1/1 -> Switch2/3
  Gain2/1 -> Divide4/2
  Demux5/4 -> [I_4]
  Demux5/3 -> [I_3]
  Demux5/5 -> [I_5]
  Demux5/2 -> [I_2]
  Demux5/1 -> [I_1]
  [Vd] -> Mux2/4
  [Ve] -> Mux2/5
  [Vc] -> Mux2/3
  [Vb] -> Mux2/2
  [Va] -> Mux2/1
  Demux3/8 -> [r23]
  Demux3/9 -> [r24]
  Demux3/10 -> [r25]
  Demux3/14 -> [r34]
  Demux3/15 -> [r35]
  Demux3/20 -> [r45]
  Constant5/1 -> Reshape1/1
  Switch2/1 -> Demux2/1, Gain2/1
  Divide4/1 -> Demux3/1
  connections:
  Simscape Component14/LConn2 -- Simscape Component9/LConn2 -- Voltage Source/RConn1 -- Simscape/LConn1 -- Simscape Component16/LConn2 -- Simscape Component7/LConn2 -- 1/RConn1 -- Simscape Component8/LConn2
  Simscape Component11/LConn2 -- Voltage Source2/RConn1 -- Simscape2/LConn1 -- Simscape Component15/RConn1 -- Simscape Component16/RConn1 -- Simscape Component1/LConn2 -- Simscape Component/LConn2 -- 3/RConn1
  Simscape Component10/LConn2 -- Voltage Source1/RConn1 -- Simscape1/LConn1 -- Simscape Component15/LConn2 -- Simscape Component14/RConn1 -- Simscape Component4/LConn2 -- Simscape Component3/LConn2 -- 2/RConn1
  Electrical Reference2/LConn1 -- Voltage Source1/RConn2
  Electrical Reference3/LConn1 -- Voltage Source2/RConn2
  Electrical Reference1/LConn1 -- Voltage Source/RConn2
  Simscape Component9/RConn1 -- gnd/LConn1
  Simscape Component9/LConn1 -- Simulink-PS Converter/RConn1
  Simscape Component10/RConn1 -- gnd1/LConn1
  Simscape Component10/LConn1 -- Simulink-PS Converter1/RConn1
  Simscape Component11/RConn1 -- gnd2/LConn1
  Simscape Component11/LConn1 -- Simulink-PS Converter2/RConn1
  Simscape Component14/LConn1 -- Simulink-PS Converter3/RConn1
  Simscape Component15/LConn1 -- Simulink-PS Converter4/RConn1
  Simscape Component16/LConn1 -- Simulink-PS Converter5/RConn1
  Simscape Component17/LConn2 -- 4/RConn1 -- Simscape Component/RConn1 -- Simscape Component3/RConn1 -- Simscape Component8/RConn1 -- Simscape Component12/LConn2 -- Voltage Source3/RConn1 -- Simscape3/LConn1
  Simscape Component12/LConn1 -- Simulink-PS Converter6/RConn1
  Simscape Component12/RConn1 -- gnd3/LConn1
  Electrical Reference4/LConn1 -- Voltage Source3/RConn2
  Simscape Component13/LConn2 -- Voltage Source4/RConn1 -- Simscape Component17/RConn1 -- Simscape Component1/RConn1 -- 5/RConn1 -- Simscape Component4/RConn1 -- Simscape Component7/RConn1 -- Simscape4/LConn1
  Simscape Component13/RConn1 -- gnd4/LConn1
  Simscape Component13/LConn1 -- Simulink-PS Converter7/RConn1
  Electrical Reference5/LConn1 -- Voltage Source4/RConn2
  Simscape Component17/LConn1 -- Simulink-PS Converter9/RConn1
  Simscape Component8/LConn1 -- Simulink-PS Converter12/RConn1
  Simscape Component7/LConn1 -- Simulink-PS Converter13/RConn1
  Simscape Component3/LConn1 -- Simulink-PS Converter15/RConn1
  Simscape Component4/LConn1 -- Simulink-PS Converter16/RConn1
  Simscape Component/LConn1 -- Simulink-PS Converter18/RConn1
  Simscape Component1/LConn1 -- Simulink-PS Converter19/RConn1

== system MATE_SynchronousMachine/MATE_LineCommutatedConverter/MATE_AGGREG/Subsystem ==
  note: yout=[ 'U_XX/Th1 ' 'U_XX/Th2 ' 'U_XX/Th3 ' 'U_XX/Th4 ' 'U_XX/Th5 ' 'U_XX/Th6 ' 'U_MATE+/vm' 'U_MATE-/vm' 'U_MATEA/vm' 'U_MATEB/vm' 'U_MATEC/vm'];
  A : PMIOPort  Side=Left
  -1 : PMIOPort  Port=2  Side=Right
  B : PMIOPort  Port=3  Side=Left
  -2 : PMIOPort  Port=4  Side=Right
  C : PMIOPort  Port=5  Side=Left
  -3 : PMIOPort  Port=6  Side=Right
  + : PMIOPort  Port=7  Side=Left
  -4 : PMIOPort  Port=8  Side=Right
  - : PMIOPort  Port=9  Side=Left
  -5 : PMIOPort  Port=10  Side=Right
  connections:
  +/RConn1 -- -1/RConn1
  -/RConn1 -- -2/RConn1
  A/RConn1 -- -3/RConn1
  B/RConn1 -- -4/RConn1
  C/RConn1 -- -5/RConn1

== system MATE_SynchronousMachine/turbine1/Hydraulic Turbine and Governor/Model ==
  wref : Inport
  Pref : Inport  Port=2
  we : Inport  Port=3
  Pe : Inport  Port=4
  dw : Inport  Port=5
  Constant1 : Constant  Value=dref
  Discrete PID Controller : Subsystem  mask(Discrete PID Controller){Kp=kp, Ki=ki, Kd=kd, TcD=td, Par_Limits=[1e6 -1e6], Init=go, Ts=Ts}
      mask prompts: Kp "Proportional gain (Kp):"; Ki "Integral gain (Ki):"; Kd "Derivative gain (Kd):"; TcD "Time constant for derivative (s):"; Par_Limits "Output limits: [ Upper   Lower ]"; Init "Output initial value:"; Ts "Sample time:"
      mask help: This block implements a discrete PID controller.
      mask init:
      | UpperLimit=Par_Limits(1);
      | LowerLimit=Par_Limits(2);
      mask Display: disp('PID');
  Sum : Sum  Inputs=+-  InputSameDT=on  SaturateOnIntegerOverflow=on  OutDataTypeStr=Inherit: Same as first input
  Sum1 : Sum  Inputs=+-  InputSameDT=on  SaturateOnIntegerOverflow=on  OutDataTypeStr=Inherit: Same as first input
  Sum5 : Sum  Inputs=-+  InputSameDT=on  SaturateOnIntegerOverflow=on  OutDataTypeStr=Inherit: Same as first input
  Switch : Switch  Threshold=0.5  SaturateOnIntegerOverflow=off
  permanent droop : Gain  Gain=Rp  SaturateOnIntegerOverflow=on  OutDataTypeStr=Inherit: Same as input  ParamDataTypeStr=Inherit: Same as input
  servo-motor : Subsystem
      mask Display: disp('servo-\nmotor')
  turbine : Subsystem
      mask Display: disp('hydraulic\nturbine')
  Pm : Outport  InitialOutput=0
  gate : Outport  Port=2  InitialOutput=0
  wires:
  Constant1/1 -> Switch/2
  Switch/1 -> permanent droop/1
  Pe/1 -> Sum5/2
  Pref/1 -> Sum5/1
  Sum1/1 -> Discrete PID Controller/1(Error)
  permanent droop/1 -> Sum1/2
  Sum/1 -> Sum1/1
  Discrete PID Controller/1(Out) -> servo-motor/1(regulator's output)
  wref/1 -> Sum/1
  we/1 -> Sum/2
  Sum5/1 -> Switch/3
  servo-motor/1(gate opening) -> turbine/2(gate opening), gate/1, Switch/1
  dw/1 -> turbine/1(dw)
  turbine/1(Pm) -> Pm/1

== system MATE_SynchronousMachine/turbine1/Mechanical model/Delay Prediction ==
  in : Inport
  F2 : Gain  Gain=2  SaturateOnIntegerOverflow=on  OutDataTypeStr=Inherit: Same as input  ParamDataTypeStr=Inherit: Same as input
  Sum1 : Sum  Inputs=+-  InputSameDT=on  SaturateOnIntegerOverflow=on  OutDataTypeStr=Inherit: Same as first input
  dw_delay : UnitDelay  SampleTime=Ts  HasFrameUpgradeWarning=on
  dw_predict : UnitDelay  SampleTime=Ts  HasFrameUpgradeWarning=on
  dw : Outport
  wires:
  dw_delay/1 -> dw_predict/1, F2/1
  in/1 -> dw_delay/1
  dw_predict/1 -> Sum1/2
  F2/1 -> Sum1/1
  Sum1/1 -> dw/1

== system MATE_SynchronousMachine/Command/Regulateur de tension (Mode automatique)/Discrete 3-phase Positive-Sequence Fundamental Value/Discrete Mean value1 ==
  note: Discrete Mean Value
  In : Inport
  Constant : Constant  Value=Vinit  SampleTime=Ts
  Discrete Variable Transport Delay : powerlib_extras/Discrete  Control Blocks/Discrete Variable Transport Delay  MaxDelay=Delay+Ts  InitialValue=0  Ts=Ts
  Gain : Gain  Gain=K1  SaturateOnIntegerOverflow=on  OutDataTypeStr=Inherit: Same as input  ParamDataTypeStr=Inherit: Same as input
  Gain1 : Gain  Gain=K2  SaturateOnIntegerOverflow=on  OutDataTypeStr=Inherit: Same as input  ParamDataTypeStr=Inherit: Same as input
  Integ4 : DiscreteIntegrator  IntegratorMethod=Integration: Trapezoidal  SampleTime=Ts  ICPrevOutput=DiscIntNeverNeededParam  ICPrevScaledInput=DiscIntNeverNeededParam
  K1 : Constant  Value=Delay  SampleTime=Ts
  K2 : Constant  Value=Freq  SampleTime=Ts
  Product : Product  InputSameDT=on  SaturateOnIntegerOverflow=on  OutDataTypeStr=Inherit: Same as first input
  Step : Step  Time=1/Freq  SampleTime=Ts
  Sum1 : Sum  Inputs=+-  InputSameDT=on  SaturateOnIntegerOverflow=on  OutDataTypeStr=Inherit: Same as first input
  Sum5 : Sum  InputSameDT=on  SaturateOnIntegerOverflow=on  OutDataTypeStr=Inherit: Same as first input
  Sum7 : Sum  Inputs=-+  InputSameDT=on  SaturateOnIntegerOverflow=on  OutDataTypeStr=Inherit: Same as first input
  Switch : Switch  Threshold=0.5  SaturateOnIntegerOverflow=off
  Unit Delay : UnitDelay  SampleTime=Ts  HasFrameUpgradeWarning=on
  Mean : Outport  VectorParamsAs1DForOutWhenUnconnected=off
  wires:
  Product/1 -> Sum5/1  "Mean value"
  Sum7/1 -> Product/1
  Integ4/1 -> Discrete Variable Transport Delay/1, Sum7/2
  K2/1 -> Product/2
  In/1 -> Integ4/1, Gain1/1, Unit Delay/1  "In"
  Sum5/1 -> Switch/1
  Step/1 -> Switch/2
  Constant/1 -> Switch/3
  Switch/1 -> Mean/1
  Discrete Variable Transport Delay/1 -> Sum7/1
  K1/1 -> Discrete Variable Transport Delay/2
  Gain1/1 -> Sum1/1
  Unit Delay/1 -> Gain/1
  Gain/1 -> Sum1/2
  Sum1/1 -> Sum5/2  "Correction"

== system MATE_SynchronousMachine/Command/Regulateur de tension (Mode automatique)/Discrete 3-phase Positive-Sequence Fundamental Value/Discrete Mean value3 ==
  note: Discrete Mean Value
  In : Inport
  Constant : Constant  Value=Vinit  SampleTime=Ts
  Discrete Variable Transport Delay : powerlib_extras/Discrete  Control Blocks/Discrete Variable Transport Delay  MaxDelay=Delay+Ts  InitialValue=0  Ts=Ts
  Gain : Gain  Gain=K1  SaturateOnIntegerOverflow=on  OutDataTypeStr=Inherit: Same as input  ParamDataTypeStr=Inherit: Same as input
  Gain1 : Gain  Gain=K2  SaturateOnIntegerOverflow=on  OutDataTypeStr=Inherit: Same as input  ParamDataTypeStr=Inherit: Same as input
  Integ4 : DiscreteIntegrator  IntegratorMethod=Integration: Trapezoidal  SampleTime=Ts  ICPrevOutput=DiscIntNeverNeededParam  ICPrevScaledInput=DiscIntNeverNeededParam
  K1 : Constant  Value=Delay  SampleTime=Ts
  K2 : Constant  Value=Freq  SampleTime=Ts
  Product : Product  InputSameDT=on  SaturateOnIntegerOverflow=on  OutDataTypeStr=Inherit: Same as first input
  Step : Step  Time=1/Freq  SampleTime=Ts
  Sum1 : Sum  Inputs=+-  InputSameDT=on  SaturateOnIntegerOverflow=on  OutDataTypeStr=Inherit: Same as first input
  Sum5 : Sum  InputSameDT=on  SaturateOnIntegerOverflow=on  OutDataTypeStr=Inherit: Same as first input
  Sum7 : Sum  Inputs=-+  InputSameDT=on  SaturateOnIntegerOverflow=on  OutDataTypeStr=Inherit: Same as first input
  Switch : Switch  Threshold=0.5  SaturateOnIntegerOverflow=off
  Unit Delay : UnitDelay  SampleTime=Ts  HasFrameUpgradeWarning=on
  Mean : Outport  VectorParamsAs1DForOutWhenUnconnected=off
  wires:
  Sum1/1 -> Sum5/2  "Correction"
  Gain/1 -> Sum1/2
  Unit Delay/1 -> Gain/1
  Gain1/1 -> Sum1/1
  K1/1 -> Discrete Variable Transport Delay/2
  Discrete Variable Transport Delay/1 -> Sum7/1
  Switch/1 -> Mean/1
  Constant/1 -> Switch/3
  Step/1 -> Switch/2
  Sum5/1 -> Switch/1
  In/1 -> Unit Delay/1, Gain1/1, Integ4/1  "In"
  K2/1 -> Product/2
  Integ4/1 -> Sum7/2, Discrete Variable Transport Delay/1
  Sum7/1 -> Product/1
  Product/1 -> Sum5/1  "Mean value"
